simulink model "CM200C_DmaCfgAndUse"  (R2013b)
settings: Solver=ode1  StartTime=0.0  StopTime=Inf  FixedStep=0.001  RelTol=1e-3
libraries: simulink x2
(part 1 of 2)
settings Model: Creator=Keyur Patel  LastModifiedBy=CZ68DS
settings OptimizationCC: BlockReduction=off  DefaultUnderspecifiedDataType=single  OptimizeBlockIOStorage=off  BufferReuse=off  ExpressionFolding=off  LocalBlockOutputs=off  OptimizeModelRefInitCode=on  LifeSpan=Inf
settings DebuggingCC: FrameProcessingCompatibilityMsg=error
settings HardwareCC: ProdIntDivRoundTo=Zero  ProdEndianess=BigEndian  ProdHWDeviceType=Generic->Custom  TargetIntDivRoundTo=Zero  TargetEndianess=BigEndian  TargetHWDeviceType=Generic->Custom
settings RTWCC: SystemTargetFile=ert.tlc  TemplateMakefile=ert_default_tmf  Description=Embedded Coder
settings CodeAppCC: IgnoreCustomStorageClasses=off
settings ERTTargetCC: CodeReplacementLibrary=C89/C90 (ANSI)  GenerateSampleERTMain=on  ERTCustomFileTemplate=example_file_process.tlc

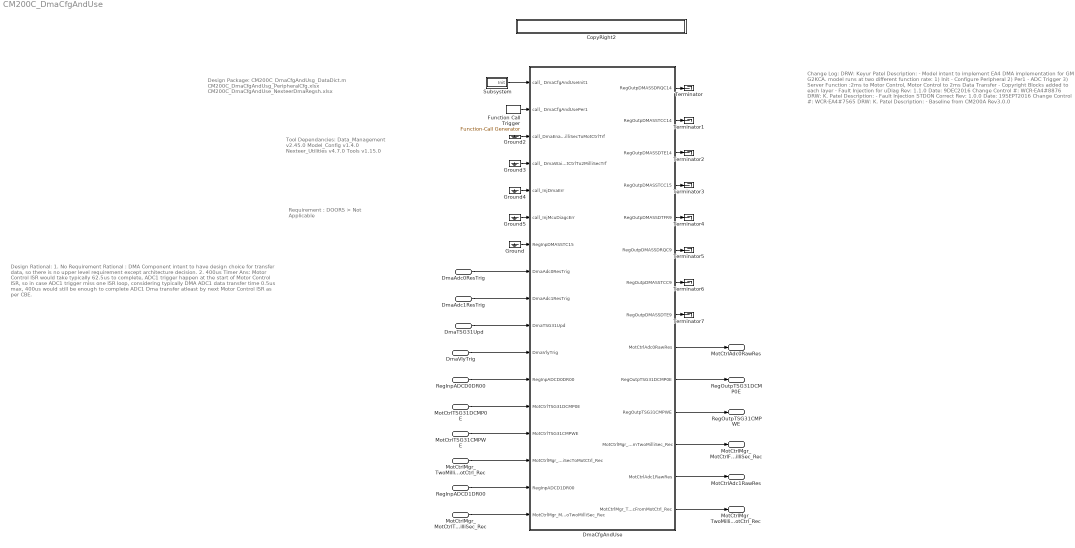
== system CM200C_DmaCfgAndUse ==
  note: Design Package:
      |
      | CM200C_DmaCfgAndUsg_DataDict.m
      | CM200C_DmaCfgAndUsg_PeripheralCfg.xlsx
      | CM200C_DmaCfgAndUse_NexteerDmaRegsh.xlsx
  note: Tool Dependancies:
      |
      | Data_Management v2.45.0
      | Model_Config v1.4.0
      | Nexteer_Utilities v4.7.0
      | Tools v1.15.0
  note: Requirement :
      |
      | DOORS > Not Applicable
  note: Change Log:
      |
      | DRW: Keyur Patel
      | Description:
      | - Model intent to implement EA4 DMA implementation for GM G2KCA.
      |    model runs at two different function rate:
      |       1) Init - Configure Peripheral
      | 	 2) Per1 - ADC Trigger
      | 	 3) Server Function :2ms to Motor Control, Motor Control to 2ms Data Transfer
      | - Copyright Blocks added to each layer
      | - Fault Injection for uDiag
      |
      | Rev: 1.1.0
      | Date: 9DEC2016
      | Change Control #: WCR-EA4#8876
      | DRW: K. Patel
      | Description:
      | - Fault Injection STDON Correct
      |
      | Rev: 1.0.0
      | Date: 19SEPT2016
      | Change Control #: WCR-EA4#7565
      | DRW: K. Patel
      | Description:
      | - Baseline from CM200A Rev3.0.0
  note: Design Rational:
      | 1. No Requirement
      | Rational :  DMA Component intent to have design choice for transfer data, so there is no upper level
      | requirement except architecture decision.
      |
      | 2. 400us Timer
      | Ans: Motor Control ISR would take typically 62.5us to complete, ADC1 trigger happen at the start of Motor
      | Control ISR, so in case ADC1  trigger miss one ISR loop, considering typically DMA ADC1 data transfer time
      | 0.5us max, 400us would still be enough to complete ADC1 Dma transfer atleast by next Motor Control
      | ISR as per CBE.
  DmaAdc0ResTrig : Inport
  DmaAdc1ResTrig : Inport  Port=2
  DmaTSG31Upd : Inport  Port=3
  DmaVlyTrig : Inport  Port=4
  RegInpADCD0DR00 : Inport  Port=5
  MotCtrlTSG31DCMP0E : Inport  Description=DMA0-3 : Source Address  Port=6
  MotCtrlTSG31CMPWE : Inport  Description=DMA0-4 : Source Address  Port=7
  MotCtrlMgr_TwoMilliSecToMotCtrl_Rec : Inport  Description=DMA1-1 : Source Address  Port=8
  RegInpADCD1DR00 : Inport  Description=DMA1-6 : Source Address  Port=9
  MotCtrlMgr_MotCtrlToTwoMilliSec_Rec : Inport  Description=DMA1-7 : Source Address  Port=10
  CopyRight2 : Subsystem  Description=|  mask(Copyright Information){none=on}
      | Copyright info block.                                               
      |                                                                     
      | Place copyright information at the top of every subsystem in design.
      mask prompts: none "No parameters"
      mask help: Place copyright information at the top of every subsystem in design.
      mask Display:
      | NxtrConf = 'Nexteer Confidential';
      | 
      | sys = bdroot; %handle for the current model ("system")
      | first = get_param(sys,'Created');
      | first = first(end-3:end);  %year is last four digits
      | 
      | last = get_param(sys,'LastModifiedDate');
      | if isempty(last)
      |     last = datestr(now,'yyyy');
      | else
      |     last = last(end-3:end);
      | end
      | 
      | if strcmp(first,last)
      |     fprintf('%s -- Copyright %s Nexteer',NxtrConf,first)
      | else
      |     fprintf('%s -- %s%s- %s Nexteer',NxtrConf,char(169),first,last)
      | end
  DmaCfgAndUse : Subsystem
  Function Call Trigger : simulink/Ports & Subsystems/Function-Call Generator  RequirementInfo="{'linktype_rmi_doors' '000089e3 (/E-STEER_New/System Specification Documents/Core Specs/Subsystem Specs/System Functions FDD/SF-46  Gross Cross Check)' '#211' 'true' 'REQ: SF046A_211' '' ; 'linktype_rmi_doors' '000089e3 (/E-STEER_New/System Specification Documents/Core Specs/Subsystem Specs/System Functions FDD/SF-46  Gross Cross Check)' '#182' 'true' 'REQ: SF046A_182' '' } %GIDa_688b36ec_1d40_4533_93c7_ec108d0c1aaf"  sample_time=0.002  numberOfIterations=1
      settings: AttributesFormatString=%<sample_time>
  Ground{,2..5} (5 alike) : Ground
  Subsystem : Subsystem
  Terminator{,1..7} (8 alike) : Terminator
  MotCtrlAdc0RawRes : Outport  Description=DMA0-1: Destination Address
  RegOutpTSG31DCMP0E : Outport  Description=DMA0-3: Destination Address  Port=2
  RegOutpTSG31CMPWE : Outport  Description=DMA0-4 : Destination Address  Port=3
  MotCtrlMgr_MotCtrlFromTwoMilliSec_Rec : Outport  Description=DMA1-1 : Destination Address  Port=4
  MotCtrlAdc1RawRes : Outport  Description=DMA1-6 : Destination Address  Port=5
  MotCtrlMgr_TwoMilliSecFromMotCtrl_Rec : Outport  Description=DMA1-7 : Destination Address  Port=6
  wires:
  Function Call Trigger/1 -> DmaCfgAndUse/2(call_ DmaCfgAndUsePer1)
  DmaCfgAndUse/1(RegOutpDMASSDRQC14) -> Terminator/1
  DmaCfgAndUse/2(RegOutpDMASSTCC14) -> Terminator1/1
  DmaCfgAndUse/3(RegOutpDMASSDTE14) -> Terminator2/1
  DmaCfgAndUse/7(RegOutpDMASSTCC9) -> Terminator6/1
  DmaCfgAndUse/6(RegOutpDMASSDRQC9) -> Terminator5/1
  DmaCfgAndUse/5(RegOutpDMASSDTFR9) -> Terminator4/1
  DmaCfgAndUse/8(RegOutpDMASSDTE9) -> Terminator7/1
  Ground/1 -> DmaCfgAndUse/7(RegInpDMASSTC15)
  DmaAdc0ResTrig/1 -> DmaCfgAndUse/8(DmaAdc0ResTrig)
  DmaAdc1ResTrig/1 -> DmaCfgAndUse/9(DmaAdc1ResTrig)
  DmaTSG31Upd/1 -> DmaCfgAndUse/10(DmaTSG31Upd)
  DmaVlyTrig/1 -> DmaCfgAndUse/11(DmaVlyTrig)
  DmaCfgAndUse/4(RegOutpDMASSTCC15) -> Terminator3/1
  RegInpADCD0DR00/1 -> DmaCfgAndUse/12(RegInpADCD0DR00)
  MotCtrlTSG31DCMP0E/1 -> DmaCfgAndUse/13(MotCtrlTSG31DCMP0E)
  MotCtrlTSG31CMPWE/1 -> DmaCfgAndUse/14(MotCtrlTSG31CMPWE)
  MotCtrlMgr_TwoMilliSecToMotCtrl_Rec/1 -> DmaCfgAndUse/15(MotCtrlMgr_TwoMilliSecToMotCtrl_Rec)
  RegInpADCD1DR00/1 -> DmaCfgAndUse/16(RegInpADCD1DR00)
  MotCtrlMgr_MotCtrlToTwoMilliSec_Rec/1 -> DmaCfgAndUse/17(MotCtrlMgr_MotCtrlToTwoMilliSec_Rec)
  DmaCfgAndUse/9(MotCtrlAdc0RawRes) -> MotCtrlAdc0RawRes/1
  DmaCfgAndUse/10(RegOutpTSG31DCMP0E) -> RegOutpTSG31DCMP0E/1
  DmaCfgAndUse/11(RegOutpTSG31CMPWE) -> RegOutpTSG31CMPWE/1
  DmaCfgAndUse/12(MotCtrlMgr_MotCtrlFromTwoMilliSec_Rec) -> MotCtrlMgr_MotCtrlFromTwoMilliSec_Rec/1
  DmaCfgAndUse/13(MotCtrlAdc1RawRes) -> MotCtrlAdc1RawRes/1
  DmaCfgAndUse/14(MotCtrlMgr_TwoMilliSecFromMotCtrl_Rec) -> MotCtrlMgr_TwoMilliSecFromMotCtrl_Rec/1
  Subsystem/1(Init) -> DmaCfgAndUse/1(call_ DmaCfgAndUseInit1)
  Ground2/1 -> DmaCfgAndUse/3(call_DmaEna2MilliSecToMotCtrlTrf)
  Ground3/1 -> DmaCfgAndUse/4(call_ DmaWaitForMotCtrlTo2MilliSecTrf)
  Ground4/1 -> DmaCfgAndUse/5(call_InjDmaErr)
  Ground5/1 -> DmaCfgAndUse/6(call_InjMcuDiagcErr)

== system CM200C_DmaCfgAndUse/CopyRight2 ==

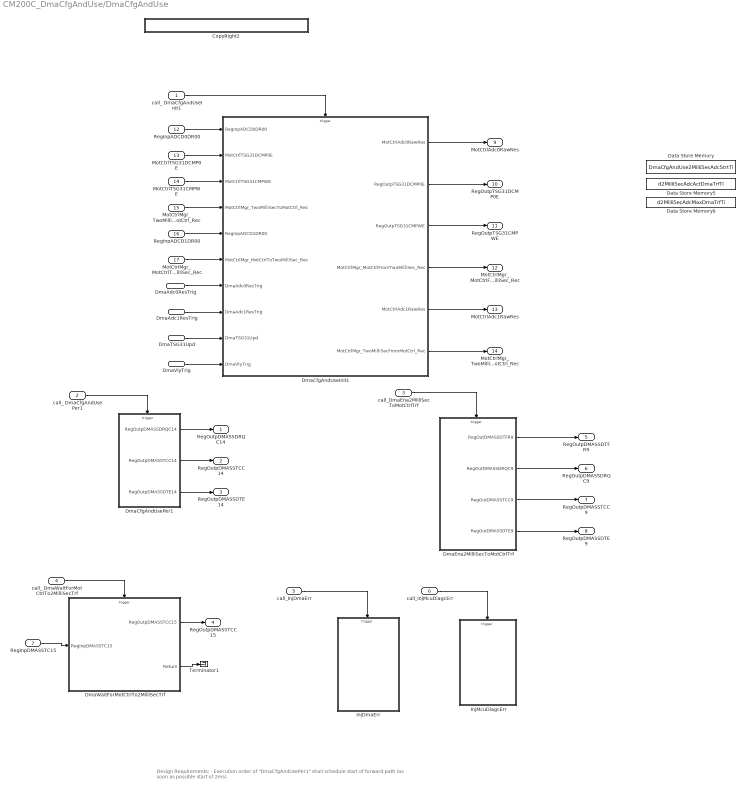
== system CM200C_DmaCfgAndUse/DmaCfgAndUse ==
  note: Design Requirements:
      |
      | - Execution order of "DmaCfgAndUsePer1" shall schedule start of forward path (as soon as possible start of 2ms).
  call_ DmaCfgAndUseInit1 : Inport
  call_ DmaCfgAndUsePer1 : Inport  Port=2
  call_DmaEna2MilliSecToMotCtrlTrf : Inport  Port=3
  call_ DmaWaitForMotCtrlTo2MilliSecTrf : Inport  Port=4
  call_InjDmaErr : Inport  Port=5
  call_InjMcuDiagcErr : Inport  Port=6
  RegInpDMASSTC15 : Inport  Port=7
  DmaAdc0ResTrig : Inport  Description=Physical Trigger : INTADCD0I3  Port=8
  DmaAdc1ResTrig : Inport  Description=Physical Trigger: INTADCD1I1  Port=9
  DmaTSG31Upd : Inport  Description=Physical Trigger: INTTSG31I11  Port=10
  DmaVlyTrig : Inport  Description=Physical Trigger: INTTSG31IVLY  Port=11
  RegInpADCD0DR00 : Inport  Port=12
  MotCtrlTSG31DCMP0E : Inport  Description=DMA0-3 : Source Address  Port=13
  MotCtrlTSG31CMPWE : Inport  Description=DMA0-4 : Source Address  Port=14
  MotCtrlMgr_TwoMilliSecToMotCtrl_Rec : Inport  Description=DMA1-1 : Source Address  Port=15
  RegInpADCD1DR00 : Inport  Description=DMA1-6 : Source Address  Port=16
  MotCtrlMgr_MotCtrlToTwoMilliSec_Rec : Inport  Description=DMA1-7 : Source Address  Port=17
  CopyRight2 : Subsystem  Description=|  mask(Copyright Information){none=on}
      | Copyright info block.                                               
      |                                                                     
      | Place copyright information at the top of every subsystem in design.
      mask prompts: none "No parameters"
      mask help: Place copyright information at the top of every subsystem in design.
      mask Display:
      | NxtrConf = 'Nexteer Confidential';
      | 
      | sys = bdroot; %handle for the current model ("system")
      | first = get_param(sys,'Created');
      | first = first(end-3:end);  %year is last four digits
      | 
      | last = get_param(sys,'LastModifiedDate');
      | if isempty(last)
      |     last = datestr(now,'yyyy');
      | else
      |     last = last(end-3:end);
      | end
      | 
      | if strcmp(first,last)
      |     fprintf('%s -- Copyright %s Nexteer',NxtrConf,first)
      | else
      |     fprintf('%s -- %s%s- %s Nexteer',NxtrConf,char(169),first,last)
      | end
  Data Store Memory : DataStoreMemory  DataStoreName=DmaCfgAndUse2MilliSecAdcStrtTi  ReadBeforeWriteMsg=warning  WriteAfterWriteMsg=warning  WriteAfterReadMsg=warning  ShowAdditionalParam=off  StateMustResolveToSignalObject=on
  Data Store Memory5 : DataStoreMemory  DataStoreName=d2MilliSecAdcActDmaTrfTi  ReadBeforeWriteMsg=warning  WriteAfterWriteMsg=warning  WriteAfterReadMsg=warning  ShowAdditionalParam=off  StateMustResolveToSignalObject=on
  Data Store Memory6 : DataStoreMemory  DataStoreName=d2MilliSecAdcMaxDmaTrfTi  ReadBeforeWriteMsg=warning  WriteAfterWriteMsg=warning  WriteAfterReadMsg=warning  ShowAdditionalParam=off  StateMustResolveToSignalObject=on
  DmaCfgAndUseInit1 : Subsystem  TreatAsAtomicUnit=on
  DmaCfgAndUsePer1 : Subsystem  TreatAsAtomicUnit=on
  DmaEna2MilliSecToMotCtrlTrf : Subsystem  TreatAsAtomicUnit=on
  DmaWaitForMotCtrlTo2MilliSecTrf : Subsystem  TreatAsAtomicUnit=on
  InjDmaErr : Subsystem  TreatAsAtomicUnit=on
  InjMcuDiagcErr : Subsystem  TreatAsAtomicUnit=on
  Terminator1 : Terminator
  RegOutpDMASSDRQC14 : Outport
  RegOutpDMASSTCC14 : Outport  Port=2
  RegOutpDMASSDTE14 : Outport  Port=3
  RegOutpDMASSTCC15 : Outport  Port=4
  RegOutpDMASSDTFR9 : Outport  Port=5
  RegOutpDMASSDRQC9 : Outport  Port=6
  RegOutpDMASSTCC9 : Outport  Port=7
  RegOutpDMASSDTE9 : Outport  Port=8
  MotCtrlAdc0RawRes : Outport  Description=DMA0-1: Destination Address  Port=9
  RegOutpTSG31DCMP0E : Outport  Description=DMA0-3: Destination Address  Port=10
  RegOutpTSG31CMPWE : Outport  Description=DMA0-4 : Destination Address  Port=11
  MotCtrlMgr_MotCtrlFromTwoMilliSec_Rec : Outport  Description=DMA1-1 : Destination Address  Port=12
  MotCtrlAdc1RawRes : Outport  Description=DMA1-6 : Destination Address  Port=13
  MotCtrlMgr_TwoMilliSecFromMotCtrl_Rec : Outport  Description=DMA1-7 : Destination Address  Port=14
  wires:
  call_ DmaCfgAndUseInit1/1 -> DmaCfgAndUseInit1/Trigger
  call_ DmaCfgAndUsePer1/1 -> DmaCfgAndUsePer1/Trigger
  call_ DmaWaitForMotCtrlTo2MilliSecTrf/1 -> DmaWaitForMotCtrlTo2MilliSecTrf/Trigger
  call_DmaEna2MilliSecToMotCtrlTrf/1 -> DmaEna2MilliSecToMotCtrlTrf/Trigger
  DmaCfgAndUsePer1/3(RegOutpDMASSDTE14) -> RegOutpDMASSDTE14/1
  DmaCfgAndUsePer1/2(RegOutpDMASSTCC14) -> RegOutpDMASSTCC14/1
  DmaCfgAndUsePer1/1(RegOutpDMASSDRQC14) -> RegOutpDMASSDRQC14/1
  DmaWaitForMotCtrlTo2MilliSecTrf/1(RegOutpDMASSTCC15) -> RegOutpDMASSTCC15/1
  DmaEna2MilliSecToMotCtrlTrf/2(RegOutDMASSDRQC9) -> RegOutpDMASSDRQC9/1
  DmaEna2MilliSecToMotCtrlTrf/4(RegOutDMASSDTE9) -> RegOutpDMASSDTE9/1
  DmaEna2MilliSecToMotCtrlTrf/3(RegOutDMASSTCC9) -> RegOutpDMASSTCC9/1
  DmaEna2MilliSecToMotCtrlTrf/1(RegOutDMASSDTFR9) -> RegOutpDMASSDTFR9/1
  RegInpDMASSTC15/1 -> DmaWaitForMotCtrlTo2MilliSecTrf/1(RegInpDMASSTC15)
  MotCtrlMgr_MotCtrlToTwoMilliSec_Rec/1 -> DmaCfgAndUseInit1/6(MotCtrlMgr_MotCtrlToTwoMilliSec_Rec)
  RegInpADCD0DR00/1 -> DmaCfgAndUseInit1/1(RegInpADCD0DR00)
  RegInpADCD1DR00/1 -> DmaCfgAndUseInit1/5(RegInpADCD1DR00)
  MotCtrlMgr_TwoMilliSecToMotCtrl_Rec/1 -> DmaCfgAndUseInit1/4(MotCtrlMgr_TwoMilliSecToMotCtrl_Rec)
  MotCtrlTSG31DCMP0E/1 -> DmaCfgAndUseInit1/2(MotCtrlTSG31DCMP0E)
  MotCtrlTSG31CMPWE/1 -> DmaCfgAndUseInit1/3(MotCtrlTSG31CMPWE)
  DmaAdc0ResTrig/1 -> DmaCfgAndUseInit1/7(DmaAdc0ResTrig)
  DmaAdc1ResTrig/1 -> DmaCfgAndUseInit1/8(DmaAdc1ResTrig)
  DmaTSG31Upd/1 -> DmaCfgAndUseInit1/9(DmaTSG31Upd)
  DmaVlyTrig/1 -> DmaCfgAndUseInit1/10(DmaVlyTrig)
  DmaWaitForMotCtrlTo2MilliSecTrf/2(Return) -> Terminator1/1
  DmaCfgAndUseInit1/1(MotCtrlAdc0RawRes) -> MotCtrlAdc0RawRes/1
  DmaCfgAndUseInit1/6(MotCtrlMgr_TwoMilliSecFromMotCtrl_Rec) -> MotCtrlMgr_TwoMilliSecFromMotCtrl_Rec/1
  DmaCfgAndUseInit1/2(RegOutpTSG31DCMP0E) -> RegOutpTSG31DCMP0E/1
  DmaCfgAndUseInit1/3(RegOutpTSG31CMPWE) -> RegOutpTSG31CMPWE/1
  DmaCfgAndUseInit1/5(MotCtrlAdc1RawRes) -> MotCtrlAdc1RawRes/1
  DmaCfgAndUseInit1/4(MotCtrlMgr_MotCtrlFromTwoMilliSec_Rec) -> MotCtrlMgr_MotCtrlFromTwoMilliSec_Rec/1
  call_InjDmaErr/1 -> InjDmaErr/Trigger
  call_InjMcuDiagcErr/1 -> InjMcuDiagcErr/Trigger

== system CM200C_DmaCfgAndUse/Subsystem ==
  CopyRight2 : Subsystem  Description=|  mask(Copyright Information){none=on}
      | Copyright info block.                                               
      |                                                                     
      | Place copyright information at the top of every subsystem in design.
      mask prompts: none "No parameters"
      mask help: Place copyright information at the top of every subsystem in design.
      mask Display:
      | NxtrConf = 'Nexteer Confidential';
      | 
      | sys = bdroot; %handle for the current model ("system")
      | first = get_param(sys,'Created');
      | first = first(end-3:end);  %year is last four digits
      | 
      | last = get_param(sys,'LastModifiedDate');
      | if isempty(last)
      |     last = datestr(now,'yyyy');
      | else
      |     last = last(end-3:end);
      | end
      | 
      | if strcmp(first,last)
      |     fprintf('%s -- Copyright %s Nexteer',NxtrConf,first)
      | else
      |     fprintf('%s -- %s%s- %s Nexteer',NxtrConf,char(169),first,last)
      | end
  Enabled Subsystem : Subsystem  TreatAsAtomicUnit=on
  Step : Step  Before=1  After=0  SampleTime=0
  Init : Outport
  wires:
  Enabled Subsystem/1(Init) -> Init/1
  Step/1 -> Enabled Subsystem/Enable

== system CM200C_DmaCfgAndUse/DmaCfgAndUse/CopyRight2 ==

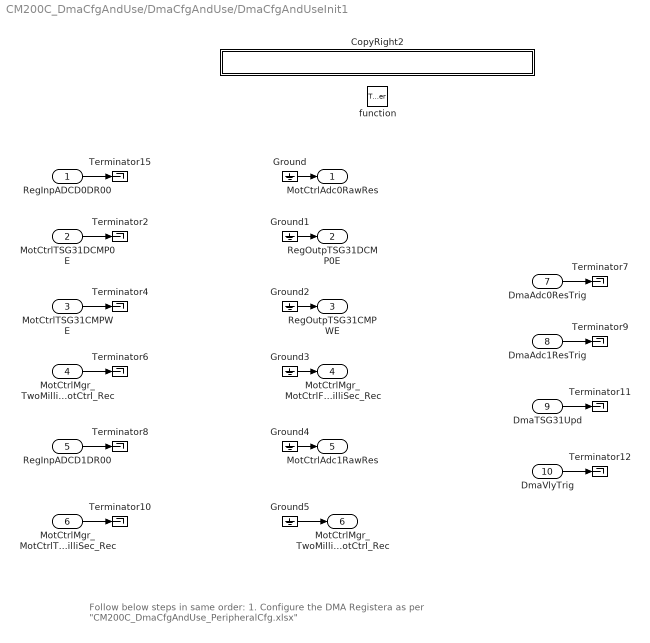
== system CM200C_DmaCfgAndUse/DmaCfgAndUse/DmaCfgAndUseInit1 ==
  note: Follow below steps in same order:
      |
      | 1. Configure the DMA Registera as per  "CM200C_DmaCfgAndUse_PeripheralCfg.xlsx"
  RegInpADCD0DR00 : Inport
      settings: AttributesFormatString=DMA0-1 : Source Address
  MotCtrlTSG31DCMP0E : Inport  Port=2
      settings: AttributesFormatString=DMA0-3 : Source Address
  MotCtrlTSG31CMPWE : Inport  Port=3
      settings: AttributesFormatString=DMA0-4 : Source Address
  MotCtrlMgr_TwoMilliSecToMotCtrl_Rec : Inport  Port=4
      settings: AttributesFormatString=DMA1-1 : Source Address
  RegInpADCD1DR00 : Inport  Port=5
      settings: AttributesFormatString=DMA1-6 : Source Address
  MotCtrlMgr_MotCtrlToTwoMilliSec_Rec : Inport  Port=6
      settings: AttributesFormatString=DMA1-7 : Source Address
  DmaAdc0ResTrig : Inport  Description=Physical Trigger : INTADCD0I3  Port=7
      settings: AttributesFormatString=%<Description>
  DmaAdc1ResTrig : Inport  Description=Physical Trigger: INTADCD1I1  Port=8
      settings: AttributesFormatString=%<Description>
  DmaTSG31Upd : Inport  Description=Physical Trigger: INTTSG31I11  Port=9
      settings: AttributesFormatString=%<Description>
  DmaVlyTrig : Inport  Description=Physical Trigger: INTTSG31VI  Port=10
      settings: AttributesFormatString=%<Description>
  function : TriggerPort  TriggerType=function-call
  CopyRight2 : Subsystem  Description=|  mask(Copyright Information){none=on}
      | Copyright info block.                                               
      |                                                                     
      | Place copyright information at the top of every subsystem in design.
      mask prompts: none "No parameters"
      mask help: Place copyright information at the top of every subsystem in design.
      mask Display:
      | NxtrConf = 'Nexteer Confidential';
      | 
      | sys = bdroot; %handle for the current model ("system")
      | first = get_param(sys,'Created');
      | first = first(end-3:end);  %year is last four digits
      | 
      | last = get_param(sys,'LastModifiedDate');
      | if isempty(last)
      |     last = datestr(now,'yyyy');
      | else
      |     last = last(end-3:end);
      | end
      | 
      | if strcmp(first,last)
      |     fprintf('%s -- Copyright %s Nexteer',NxtrConf,first)
      | else
      |     fprintf('%s -- %s%s- %s Nexteer',NxtrConf,char(169),first,last)
      | end
  Ground{,1..5} (6 alike) : Ground
  Terminator{2,4,6..12,15} (10 alike) : Terminator
  MotCtrlAdc0RawRes : Outport  Description=DMA0-1: Destination Address
      settings: AttributesFormatString=%<Description>
  RegOutpTSG31DCMP0E : Outport  Description=DMA0-3: Destination Address  Port=2
      settings: AttributesFormatString=%<Description>
  RegOutpTSG31CMPWE : Outport  Description=DMA0-4 : Destination Address  Port=3
      settings: AttributesFormatString=%<Description>
  MotCtrlMgr_MotCtrlFromTwoMilliSec_Rec : Outport  Description=DMA1-1 : Destination Address  Port=4
      settings: AttributesFormatString=%<Description>
  MotCtrlAdc1RawRes : Outport  Description=DMA1-6 : Destination Address  Port=5
      settings: AttributesFormatString=%<Description>
  MotCtrlMgr_TwoMilliSecFromMotCtrl_Rec : Outport  Description=DMA1-7 : Destination Address  Port=6
      settings: AttributesFormatString=%<Description>
  wires:
  RegInpADCD0DR00/1 -> Terminator15/1
  MotCtrlTSG31DCMP0E/1 -> Terminator2/1
  MotCtrlTSG31CMPWE/1 -> Terminator4/1
  MotCtrlMgr_TwoMilliSecToMotCtrl_Rec/1 -> Terminator6/1
  RegInpADCD1DR00/1 -> Terminator8/1
  MotCtrlMgr_MotCtrlToTwoMilliSec_Rec/1 -> Terminator10/1
  Ground/1 -> MotCtrlAdc0RawRes/1
  Ground1/1 -> RegOutpTSG31DCMP0E/1
  Ground2/1 -> RegOutpTSG31CMPWE/1
  Ground3/1 -> MotCtrlMgr_MotCtrlFromTwoMilliSec_Rec/1
  Ground4/1 -> MotCtrlAdc1RawRes/1
  Ground5/1 -> MotCtrlMgr_TwoMilliSecFromMotCtrl_Rec/1
  DmaAdc0ResTrig/1 -> Terminator7/1
  DmaAdc1ResTrig/1 -> Terminator9/1
  DmaTSG31Upd/1 -> Terminator11/1
  DmaVlyTrig/1 -> Terminator12/1

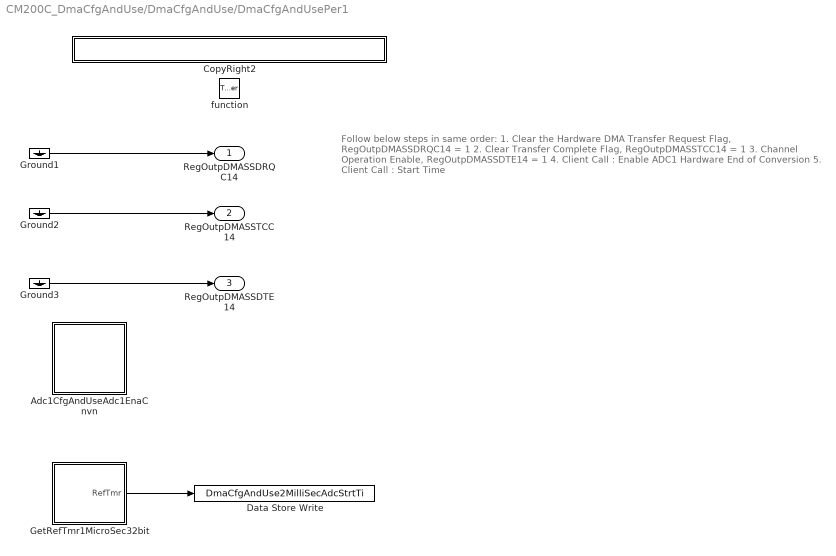
== system CM200C_DmaCfgAndUse/DmaCfgAndUse/DmaCfgAndUsePer1 ==
  note: Follow below steps in same order:
      |
      | 1. Clear the Hardware DMA Transfer Request Flag, RegOutpDMASSDRQC14 = 1
      | 2. Clear Transfer Complete Flag, RegOutpDMASSTCC14 = 1
      | 3. Channel Operation Enable, RegOutpDMASSDTE14 = 1
      | 4. Client Call : Enable ADC1 Hardware End of Conversion
      | 5. Client Call : Start Time
  function : TriggerPort  TriggerType=function-call
  Adc1CfgAndUseAdc1EnaCnvn : Subsystem
      settings: AttributesFormatString=Client Call : Enable ADC1 Hardware End of Conversion
  CopyRight2 : Subsystem  Description=|  mask(Copyright Information){none=on}
      | Copyright info block.                                               
      |                                                                     
      | Place copyright information at the top of every subsystem in design.
      mask prompts: none "No parameters"
      mask help: Place copyright information at the top of every subsystem in design.
      mask Display:
      | NxtrConf = 'Nexteer Confidential';
      | 
      | sys = bdroot; %handle for the current model ("system")
      | first = get_param(sys,'Created');
      | first = first(end-3:end);  %year is last four digits
      | 
      | last = get_param(sys,'LastModifiedDate');
      | if isempty(last)
      |     last = datestr(now,'yyyy');
      | else
      |     last = last(end-3:end);
      | end
      | 
      | if strcmp(first,last)
      |     fprintf('%s -- Copyright %s Nexteer',NxtrConf,first)
      | else
      |     fprintf('%s -- %s%s- %s Nexteer',NxtrConf,char(169),first,last)
      | end
  Data Store Write : DataStoreWrite  DataStoreName=DmaCfgAndUse2MilliSecAdcStrtTi
  GetRefTmr1MicroSec32bit : Subsystem
      settings: AttributesFormatString=Client Call : Start Time
  Ground1 : Ground
  Ground2 : Ground
  Ground3 : Ground
  RegOutpDMASSDRQC14 : Outport
  RegOutpDMASSTCC14 : Outport  Port=2
  RegOutpDMASSDTE14 : Outport  Port=3
  wires:
  Ground1/1 -> RegOutpDMASSDRQC14/1
  Ground2/1 -> RegOutpDMASSTCC14/1
  Ground3/1 -> RegOutpDMASSDTE14/1
  GetRefTmr1MicroSec32bit/1(RefTmr) -> Data Store Write/1

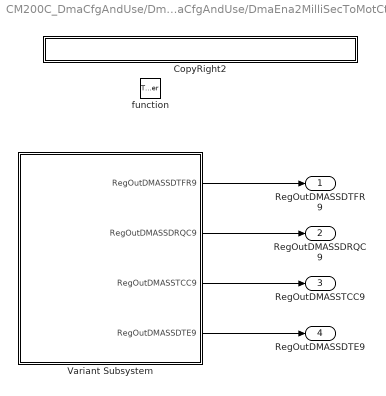
== system CM200C_DmaCfgAndUse/DmaCfgAndUse/DmaEna2MilliSecToMotCtrlTrf ==
  function : TriggerPort  TriggerType=function-call
  CopyRight2 : Subsystem  Description=|  mask(Copyright Information){none=on}
      | Copyright info block.                                               
      |                                                                     
      | Place copyright information at the top of every subsystem in design.
      mask prompts: none "No parameters"
      mask help: Place copyright information at the top of every subsystem in design.
      mask Display:
      | NxtrConf = 'Nexteer Confidential';
      | 
      | sys = bdroot; %handle for the current model ("system")
      | first = get_param(sys,'Created');
      | first = first(end-3:end);  %year is last four digits
      | 
      | last = get_param(sys,'LastModifiedDate');
      | if isempty(last)
      |     last = datestr(now,'yyyy');
      | else
      |     last = last(end-3:end);
      | end
      | 
      | if strcmp(first,last)
      |     fprintf('%s -- Copyright %s Nexteer',NxtrConf,first)
      | else
      |     fprintf('%s -- %s%s- %s Nexteer',NxtrConf,char(169),first,last)
      | end
  Variant Subsystem : Subsystem  Variant=on
      settings: AttributesFormatString=%<VariantControl>
  RegOutDMASSDTFR9 : Outport
  RegOutDMASSDRQC9 : Outport  Port=2
  RegOutDMASSTCC9 : Outport  Port=3
  RegOutDMASSDTE9 : Outport  Port=4
  wires:
  Variant Subsystem/2(RegOutDMASSDRQC9) -> RegOutDMASSDRQC9/1
  Variant Subsystem/1(RegOutDMASSDTFR9) -> RegOutDMASSDTFR9/1
  Variant Subsystem/3(RegOutDMASSTCC9) -> RegOutDMASSTCC9/1
  Variant Subsystem/4(RegOutDMASSDTE9) -> RegOutDMASSDTE9/1

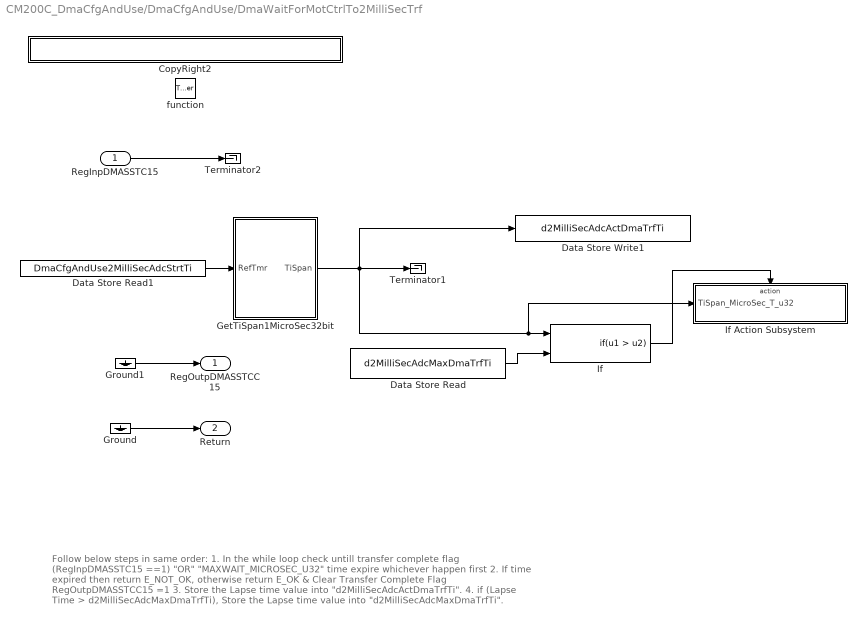
== system CM200C_DmaCfgAndUse/DmaCfgAndUse/DmaWaitForMotCtrlTo2MilliSecTrf ==
  note: Follow below steps in same order:
      |
      | 1. In the while loop check untill transfer complete flag (RegInpDMASSTC15 ==1) "OR" "MAXWAIT_MICROSEC_U32" time expire whichever happen first
      | 2. If time expired then return E_NOT_OK,
      |     otherwise return E_OK & Clear Transfer Complete Flag RegOutpDMASSTCC15 =1
      | 3. Store the Lapse time value into "d2MilliSecAdcActDmaTrfTi".
      | 4. if (Lapse Time > d2MilliSecAdcMaxDmaTrfTi), Store the Lapse time value into "d2MilliSecAdcMaxDmaTrfTi".
  RegInpDMASSTC15 : Inport
      settings: AttributesFormatString=Transfer Complete Flag Status Check
  function : TriggerPort  TriggerType=function-call
  CopyRight2 : Subsystem  Description=|  mask(Copyright Information){none=on}
      | Copyright info block.                                               
      |                                                                     
      | Place copyright information at the top of every subsystem in design.
      mask prompts: none "No parameters"
      mask help: Place copyright information at the top of every subsystem in design.
      mask Display:
      | NxtrConf = 'Nexteer Confidential';
      | 
      | sys = bdroot; %handle for the current model ("system")
      | first = get_param(sys,'Created');
      | first = first(end-3:end);  %year is last four digits
      | 
      | last = get_param(sys,'LastModifiedDate');
      | if isempty(last)
      |     last = datestr(now,'yyyy');
      | else
      |     last = last(end-3:end);
      | end
      | 
      | if strcmp(first,last)
      |     fprintf('%s -- Copyright %s Nexteer',NxtrConf,first)
      | else
      |     fprintf('%s -- %s%s- %s Nexteer',NxtrConf,char(169),first,last)
      | end
  Data Store Read : DataStoreRead  DataStoreName=d2MilliSecAdcMaxDmaTrfTi
  Data Store Read1 : DataStoreRead  DataStoreName=DmaCfgAndUse2MilliSecAdcStrtTi
  Data Store Write1 : DataStoreWrite  DataStoreName=d2MilliSecAdcActDmaTrfTi
  GetTiSpan1MicroSec32bit : Subsystem
  Ground : Ground
  Ground1 : Ground
  If : If  NumInputs=2  IfExpression=u1 > u2  ShowElse=off
  If Action Subsystem : Subsystem  TreatAsAtomicUnit=on
  Terminator1 : Terminator
      settings: Description=TiSpan_MicroSec_T_u32  AttributesFormatString=%<Description>
  Terminator2 : Terminator
  RegOutpDMASSTCC15 : Outport
  Return : Outport  Port=2
  wires:
  Ground1/1 -> RegOutpDMASSTCC15/1
  RegInpDMASSTC15/1 -> Terminator2/1
  Ground/1 -> Return/1
  Data Store Read1/1 -> GetTiSpan1MicroSec32bit/1(RefTmr)
  GetTiSpan1MicroSec32bit/1(TiSpan) -> Data Store Write1/1, If Action Subsystem/1(TiSpan_MicroSec_T_u32), If/1, Terminator1/1
  If/1 -> If Action Subsystem/Action
  Data Store Read/1 -> If/2

== system CM200C_DmaCfgAndUse/DmaCfgAndUse/InjDmaErr ==
  function : TriggerPort  TriggerType=function-call
  CopyRight2 : Subsystem  Description=|  mask(Copyright Information){none=on}
      | Copyright info block.                                               
      |                                                                     
      | Place copyright information at the top of every subsystem in design.
      mask prompts: none "No parameters"
      mask help: Place copyright information at the top of every subsystem in design.
      mask Display:
      | NxtrConf = 'Nexteer Confidential';
      | 
      | sys = bdroot; %handle for the current model ("system")
      | first = get_param(sys,'Created');
      | first = first(end-3:end);  %year is last four digits
      | 
      | last = get_param(sys,'LastModifiedDate');
      | if isempty(last)
      |     last = datestr(now,'yyyy');
      | else
      |     last = last(end-3:end);
      | end
      | 
      | if strcmp(first,last)
      |     fprintf('%s -- Copyright %s Nexteer',NxtrConf,first)
      | else
      |     fprintf('%s -- %s%s- %s Nexteer',NxtrConf,char(169),first,last)
      | end
  Variant Subsystem : Subsystem  Variant=on

== system CM200C_DmaCfgAndUse/DmaCfgAndUse/InjMcuDiagcErr ==
  function : TriggerPort  TriggerType=function-call
  CopyRight2 : Subsystem  Description=|  mask(Copyright Information){none=on}
      | Copyright info block.                                               
      |                                                                     
      | Place copyright information at the top of every subsystem in design.
      mask prompts: none "No parameters"
      mask help: Place copyright information at the top of every subsystem in design.
      mask Display:
      | NxtrConf = 'Nexteer Confidential';
      | 
      | sys = bdroot; %handle for the current model ("system")
      | first = get_param(sys,'Created');
      | first = first(end-3:end);  %year is last four digits
      | 
      | last = get_param(sys,'LastModifiedDate');
      | if isempty(last)
      |     last = datestr(now,'yyyy');
      | else
      |     last = last(end-3:end);
      | end
      | 
      | if strcmp(first,last)
      |     fprintf('%s -- Copyright %s Nexteer',NxtrConf,first)
      | else
      |     fprintf('%s -- %s%s- %s Nexteer',NxtrConf,char(169),first,last)
      | end
  Variant Subsystem : Subsystem  Variant=on

== system CM200C_DmaCfgAndUse/Subsystem/CopyRight2 ==

== system CM200C_DmaCfgAndUse/Subsystem/Enabled Subsystem ==
  Enable : EnablePort
  CopyRight2 : Subsystem  Description=|  mask(Copyright Information){none=on}
      | Copyright info block.                                               
      |                                                                     
      | Place copyright information at the top of every subsystem in design.
      mask prompts: none "No parameters"
      mask help: Place copyright information at the top of every subsystem in design.
      mask Display:
      | NxtrConf = 'Nexteer Confidential';
      | 
      | sys = bdroot; %handle for the current model ("system")
      | first = get_param(sys,'Created');
      | first = first(end-3:end);  %year is last four digits
      | 
      | last = get_param(sys,'LastModifiedDate');
      | if isempty(last)
      |     last = datestr(now,'yyyy');
      | else
      |     last = last(end-3:end);
      | end
      | 
      | if strcmp(first,last)
      |     fprintf('%s -- Copyright %s Nexteer',NxtrConf,first)
      | else
      |     fprintf('%s -- %s%s- %s Nexteer',NxtrConf,char(169),first,last)
      | end
  Function Call Trigger : simulink/Ports & Subsystems/Function-Call Generator  RequirementInfo="{'linktype_rmi_doors' '000089e3 (/E-STEER_New/System Specification Documents/Core Specs/Subsystem Specs/System Functions FDD/SF-46  Gross Cross Check)' '#211' 'true' 'REQ: SF046A_211' '' ; 'linktype_rmi_doors' '000089e3 (/E-STEER_New/System Specification Documents/Core Specs/Subsystem Specs/System Functions FDD/SF-46  Gross Cross Check)' '#182' 'true' 'REQ: SF046A_182' '' } %GIDa_cf5bacff_48a9_4312_b446_700ab36e3d94"  sample_time=0.002  numberOfIterations=1
      settings: AttributesFormatString=%<sample_time>
  Init : Outport
  wires:
  Function Call Trigger/1 -> Init/1

== system CM200C_DmaCfgAndUse/DmaCfgAndUse/DmaCfgAndUseInit1/CopyRight2 ==

== system CM200C_DmaCfgAndUse/DmaCfgAndUse/DmaCfgAndUsePer1/Adc1CfgAndUseAdc1EnaCnvn ==
  CopyRight2 : Subsystem  Description=|  mask(Copyright Information){none=on}
      | Copyright info block.                                               
      |                                                                     
      | Place copyright information at the top of every subsystem in design.
      mask prompts: none "No parameters"
      mask help: Place copyright information at the top of every subsystem in design.
      mask Display:
      | NxtrConf = 'Nexteer Confidential';
      | 
      | sys = bdroot; %handle for the current model ("system")
      | first = get_param(sys,'Created');
      | first = first(end-3:end);  %year is last four digits
      | 
      | last = get_param(sys,'LastModifiedDate');
      | if isempty(last)
      |     last = datestr(now,'yyyy');
      | else
      |     last = last(end-3:end);
      | end
      | 
      | if strcmp(first,last)
      |     fprintf('%s -- Copyright %s Nexteer',NxtrConf,first)
      | else
      |     fprintf('%s -- %s%s- %s Nexteer',NxtrConf,char(169),first,last)
      | end

== system CM200C_DmaCfgAndUse/DmaCfgAndUse/DmaCfgAndUsePer1/CopyRight2 ==

== system CM200C_DmaCfgAndUse/DmaCfgAndUse/DmaCfgAndUsePer1/GetRefTmr1MicroSec32bit ==
  CopyRight2 : Subsystem  Description=|  mask(Copyright Information){none=on}
      | Copyright info block.                                               
      |                                                                     
      | Place copyright information at the top of every subsystem in design.
      mask prompts: none "No parameters"
      mask help: Place copyright information at the top of every subsystem in design.
      mask Display:
      | NxtrConf = 'Nexteer Confidential';
      | 
      | sys = bdroot; %handle for the current model ("system")
      | first = get_param(sys,'Created');
      | first = first(end-3:end);  %year is last four digits
      | 
      | last = get_param(sys,'LastModifiedDate');
      | if isempty(last)
      |     last = datestr(now,'yyyy');
      | else
      |     last = last(end-3:end);
      | end
      | 
      | if strcmp(first,last)
      |     fprintf('%s -- Copyright %s Nexteer',NxtrConf,first)
      | else
      |     fprintf('%s -- %s%s- %s Nexteer',NxtrConf,char(169),first,last)
      | end
  Ground : Ground
  RefTmr : Outport
  wires:
  Ground/1 -> RefTmr/1

== system CM200C_DmaCfgAndUse/DmaCfgAndUse/DmaEna2MilliSecToMotCtrlTrf/CopyRight2 ==

== system CM200C_DmaCfgAndUse/DmaCfgAndUse/DmaEna2MilliSecToMotCtrlTrf/Variant Subsystem ==
  note: 1) Add Subsystem or Model blocks as valid variant choices.
      | 2) You cannot connect blocks at this level. At simulation, connectivity is automatically
      | determined, based on the active variant and port name matching.
  ErrInj : Subsystem  VariantControl=MCUDIAGCERRINJ == STD_ON
  NoErrInj : Subsystem  VariantControl=MCUDIAGCERRINJ == STD_OFF
  RegOutDMASSDTFR9 : Outport
  RegOutDMASSDRQC9 : Outport  Port=2
  RegOutDMASSTCC9 : Outport  Port=3
  RegOutDMASSDTE9 : Outport  Port=4

== system CM200C_DmaCfgAndUse/DmaCfgAndUse/DmaWaitForMotCtrlTo2MilliSecTrf/CopyRight2 ==

== system CM200C_DmaCfgAndUse/DmaCfgAndUse/DmaWaitForMotCtrlTo2MilliSecTrf/GetTiSpan1MicroSec32bit ==
  RefTmr : Inport
  CopyRight2 : Subsystem  Description=|  mask(Copyright Information){none=on}
      | Copyright info block.                                               
      |                                                                     
      | Place copyright information at the top of every subsystem in design.
      mask prompts: none "No parameters"
      mask help: Place copyright information at the top of every subsystem in design.
      mask Display:
      | NxtrConf = 'Nexteer Confidential';
      | 
      | sys = bdroot; %handle for the current model ("system")
      | first = get_param(sys,'Created');
      | first = first(end-3:end);  %year is last four digits
      | 
      | last = get_param(sys,'LastModifiedDate');
      | if isempty(last)
      |     last = datestr(now,'yyyy');
      | else
      |     last = last(end-3:end);
      | end
      | 
      | if strcmp(first,last)
      |     fprintf('%s -- Copyright %s Nexteer',NxtrConf,first)
      | else
      |     fprintf('%s -- %s%s- %s Nexteer',NxtrConf,char(169),first,last)
      | end
  Ground : Ground
  TiSpan : Outport
  wires:
  Ground/1 -> TiSpan/1

== system CM200C_DmaCfgAndUse/DmaCfgAndUse/DmaWaitForMotCtrlTo2MilliSecTrf/If Action Subsystem ==
  TiSpan_MicroSec_T_u32 : Inport
  Action Port : ActionPort  ActionType=then
  CopyRight2 : Subsystem  Description=|  mask(Copyright Information){none=on}
      | Copyright info block.                                               
      |                                                                     
      | Place copyright information at the top of every subsystem in design.
      mask prompts: none "No parameters"
      mask help: Place copyright information at the top of every subsystem in design.
      mask Display:
      | NxtrConf = 'Nexteer Confidential';
      | 
      | sys = bdroot; %handle for the current model ("system")
      | first = get_param(sys,'Created');
      | first = first(end-3:end);  %year is last four digits
      | 
      | last = get_param(sys,'LastModifiedDate');
      | if isempty(last)
      |     last = datestr(now,'yyyy');
      | else
      |     last = last(end-3:end);
      | end
      | 
      | if strcmp(first,last)
      |     fprintf('%s -- Copyright %s Nexteer',NxtrConf,first)
      | else
      |     fprintf('%s -- %s%s- %s Nexteer',NxtrConf,char(169),first,last)
      | end
  Data Store Write : DataStoreWrite  DataStoreName=d2MilliSecAdcMaxDmaTrfTi
  wires:
  TiSpan_MicroSec_T_u32/1 -> Data Store Write/1

== system CM200C_DmaCfgAndUse/DmaCfgAndUse/InjDmaErr/CopyRight2 ==

== system CM200C_DmaCfgAndUse/DmaCfgAndUse/InjDmaErr/Variant Subsystem ==
  note: 1) Add Subsystem or Model blocks as valid variant choices.
      | 2) You cannot connect blocks at this level. At simulation, connectivity is automatically
      | determined, based on the active variant and port name matching.
  ErrInj : Subsystem  VariantControl=MCUDIAGCERRINJ == STD_ON

== system CM200C_DmaCfgAndUse/DmaCfgAndUse/InjMcuDiagcErr/CopyRight2 ==

== system CM200C_DmaCfgAndUse/DmaCfgAndUse/InjMcuDiagcErr/Variant Subsystem ==
  note: 1) Add Subsystem or Model blocks as valid variant choices.
      | 2) You cannot connect blocks at this level. At simulation, connectivity is automatically
      | determined, based on the active variant and port name matching.
  ErrInj : Subsystem  VariantControl=MCUDIAGCERRINJ == STD_ON

== system CM200C_DmaCfgAndUse/Subsystem/Enabled Subsystem/CopyRight2 ==

== system CM200C_DmaCfgAndUse/DmaCfgAndUse/DmaCfgAndUsePer1/Adc1CfgAndUseAdc1EnaCnvn/CopyRight2 ==

== system CM200C_DmaCfgAndUse/DmaCfgAndUse/DmaCfgAndUsePer1/GetRefTmr1MicroSec32bit/CopyRight2 ==

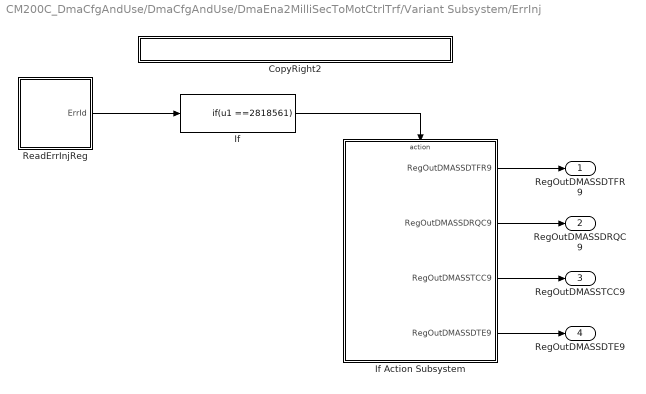
== system CM200C_DmaCfgAndUse/DmaCfgAndUse/DmaEna2MilliSecToMotCtrlTrf/Variant Subsystem/ErrInj ==
  CopyRight2 : Subsystem  Description=|  mask(Copyright Information){none=on}
      | Copyright info block.                                               
      |                                                                     
      | Place copyright information at the top of every subsystem in design.
      mask prompts: none "No parameters"
      mask help: Place copyright information at the top of every subsystem in design.
      mask Display:
      | NxtrConf = 'Nexteer Confidential';
      | 
      | sys = bdroot; %handle for the current model ("system")
      | first = get_param(sys,'Created');
      | first = first(end-3:end);  %year is last four digits
      | 
      | last = get_param(sys,'LastModifiedDate');
      | if isempty(last)
      |     last = datestr(now,'yyyy');
      | else
      |     last = last(end-3:end);
      | end
      | 
      | if strcmp(first,last)
      |     fprintf('%s -- Copyright %s Nexteer',NxtrConf,first)
      | else
      |     fprintf('%s -- %s%s- %s Nexteer',NxtrConf,char(169),first,last)
      | end
  If : If  Description=Err ID - 0x002B0201  IfExpression=u1 ==2818561  ShowElse=off
      settings: AttributesFormatString=|
      | %<IfExpression>
      | %<Description>
  If Action Subsystem : Subsystem  TreatAsAtomicUnit=on
  ReadErrInjReg : Subsystem
      settings: AttributesFormatString=Client Call : Read the Fault Injection Register
  RegOutDMASSDTFR9 : Outport
  RegOutDMASSDRQC9 : Outport  Port=2
  RegOutDMASSTCC9 : Outport  Port=3
  RegOutDMASSDTE9 : Outport  Port=4
  wires:
  ReadErrInjReg/1(ErrId) -> If/1
  If/1 -> If Action Subsystem/Action
  If Action Subsystem/3(RegOutDMASSTCC9) -> RegOutDMASSTCC9/1
  If Action Subsystem/1(RegOutDMASSDTFR9) -> RegOutDMASSDTFR9/1
  If Action Subsystem/2(RegOutDMASSDRQC9) -> RegOutDMASSDRQC9/1
  If Action Subsystem/4(RegOutDMASSDTE9) -> RegOutDMASSDTE9/1

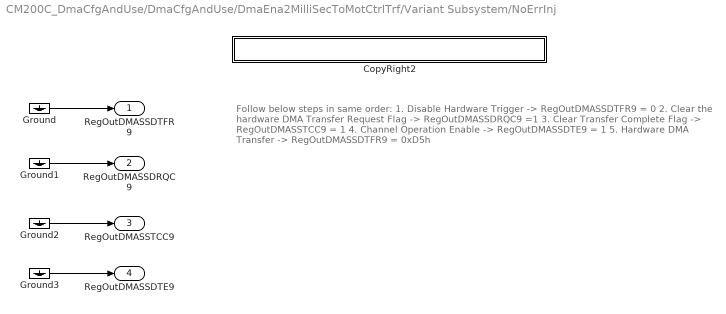
== system CM200C_DmaCfgAndUse/DmaCfgAndUse/DmaEna2MilliSecToMotCtrlTrf/Variant Subsystem/NoErrInj ==
  note: Follow below steps in same order:
      |
      | 1. Disable Hardware Trigger -> RegOutDMASSDTFR9 = 0
      | 2. Clear the hardware DMA Transfer Request Flag -> RegOutDMASSDRQC9 =1
      | 3. Clear Transfer Complete Flag -> RegOutDMASSTCC9 = 1
      | 4. Channel Operation Enable -> RegOutDMASSDTE9 = 1
      | 5. Hardware DMA Transfer -> RegOutDMASSDTFR9 = 0xD5h
  CopyRight2 : Subsystem  Description=|  mask(Copyright Information){none=on}
      | Copyright info block.                                               
      |                                                                     
      | Place copyright information at the top of every subsystem in design.
      mask prompts: none "No parameters"
      mask help: Place copyright information at the top of every subsystem in design.
      mask Display:
      | NxtrConf = 'Nexteer Confidential';
      | 
      | sys = bdroot; %handle for the current model ("system")
      | first = get_param(sys,'Created');
      | first = first(end-3:end);  %year is last four digits
      | 
      | last = get_param(sys,'LastModifiedDate');
      | if isempty(last)
      |     last = datestr(now,'yyyy');
      | else
      |     last = last(end-3:end);
      | end
      | 
      | if strcmp(first,last)
      |     fprintf('%s -- Copyright %s Nexteer',NxtrConf,first)
      | else
      |     fprintf('%s -- %s%s- %s Nexteer',NxtrConf,char(169),first,last)
      | end
  Ground{,1..3} (4 alike) : Ground
  RegOutDMASSDTFR9 : Outport
  RegOutDMASSDRQC9 : Outport  Port=2
  RegOutDMASSTCC9 : Outport  Port=3
  RegOutDMASSDTE9 : Outport  Port=4
  wires:
  Ground3/1 -> RegOutDMASSDTE9/1
  Ground2/1 -> RegOutDMASSTCC9/1
  Ground1/1 -> RegOutDMASSDRQC9/1
  Ground/1 -> RegOutDMASSDTFR9/1

== system CM200C_DmaCfgAndUse/DmaCfgAndUse/DmaWaitForMotCtrlTo2MilliSecTrf/GetTiSpan1MicroSec32bit/CopyRight2 ==

== system CM200C_DmaCfgAndUse/DmaCfgAndUse/DmaWaitForMotCtrlTo2MilliSecTrf/If Action Subsystem/CopyRight2 ==

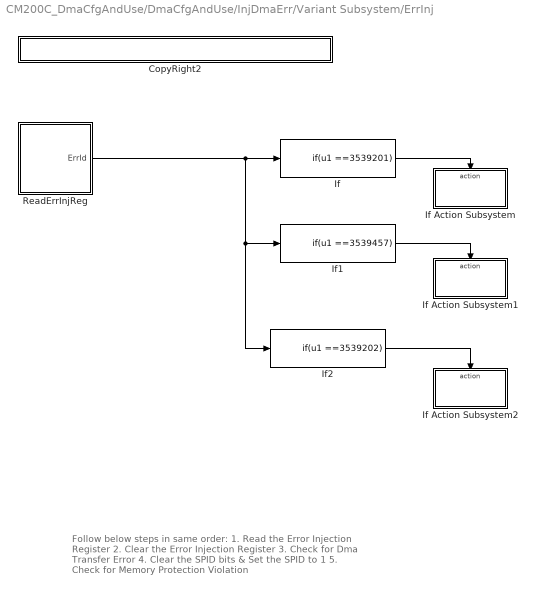
== system CM200C_DmaCfgAndUse/DmaCfgAndUse/InjDmaErr/Variant Subsystem/ErrInj ==
  note: Follow below steps in same order:
      |
      | 1. Read the Error Injection Register
      | 2. Clear the Error Injection Register
      | 3. Check for Dma Transfer Error
      | 4. Clear the SPID bits & Set the SPID to 1
      | 5. Check for Memory Protection Violation
  CopyRight2 : Subsystem  Description=|  mask(Copyright Information){none=on}
      | Copyright info block.                                               
      |                                                                     
      | Place copyright information at the top of every subsystem in design.
      mask prompts: none "No parameters"
      mask help: Place copyright information at the top of every subsystem in design.
      mask Display:
      | NxtrConf = 'Nexteer Confidential';
      | 
      | sys = bdroot; %handle for the current model ("system")
      | first = get_param(sys,'Created');
      | first = first(end-3:end);  %year is last four digits
      | 
      | last = get_param(sys,'LastModifiedDate');
      | if isempty(last)
      |     last = datestr(now,'yyyy');
      | else
      |     last = last(end-3:end);
      | end
      | 
      | if strcmp(first,last)
      |     fprintf('%s -- Copyright %s Nexteer',NxtrConf,first)
      | else
      |     fprintf('%s -- %s%s- %s Nexteer',NxtrConf,char(169),first,last)
      | end
  If : If  Description=ErrId - 0x00360101  IfExpression=u1 ==3539201  ShowElse=off
      settings: AttributesFormatString=|
      | %<IfExpression>
      | %<Description>
  If Action Subsystem : Subsystem  TreatAsAtomicUnit=on
  If Action Subsystem1 : Subsystem  TreatAsAtomicUnit=on
  If Action Subsystem2 : Subsystem  TreatAsAtomicUnit=on
  If1 : If  Description=ErrId - 0x00360201  IfExpression=u1 ==3539457  ShowElse=off
      settings: AttributesFormatString=|
      | %<IfExpression>
      | %<Description>
  If2 : If  Description=ErrId - 0x00360102  IfExpression=u1 ==3539202  ShowElse=off
      settings: AttributesFormatString=|
      | %<IfExpression>
      | %<Description>
  ReadErrInjReg : Subsystem
      settings: AttributesFormatString=Client Call : Read the Fault Injection Register
  wires:
  ReadErrInjReg/1(ErrId) -> If2/1, If1/1, If/1
  If/1 -> If Action Subsystem/Action
  If1/1 -> If Action Subsystem1/Action
  If2/1 -> If Action Subsystem2/Action

== system CM200C_DmaCfgAndUse/DmaCfgAndUse/InjMcuDiagcErr/Variant Subsystem/ErrInj ==
  note: Follow below steps in same order:
      |
      | 1. Read the Error Injection Register
      | 2. Check for Dma Transfer Error
      |    2a. Clear the Error Injection Register
      |    2b. Clear the DMASSDCEN15
  Action : Subsystem  TreatAsAtomicUnit=on
  CopyRight2 : Subsystem  Description=|  mask(Copyright Information){none=on}
      | Copyright info block.                                               
      |                                                                     
      | Place copyright information at the top of every subsystem in design.
      mask prompts: none "No parameters"
      mask help: Place copyright information at the top of every subsystem in design.
      mask Display:
      | NxtrConf = 'Nexteer Confidential';
      | 
      | sys = bdroot; %handle for the current model ("system")
      | first = get_param(sys,'Created');
      | first = first(end-3:end);  %year is last four digits
      | 
      | last = get_param(sys,'LastModifiedDate');
      | if isempty(last)
      |     last = datestr(now,'yyyy');
      | else
      |     last = last(end-3:end);
      | end
      | 
      | if strcmp(first,last)
      |     fprintf('%s -- Copyright %s Nexteer',NxtrConf,first)
      | else
      |     fprintf('%s -- %s%s- %s Nexteer',NxtrConf,char(169),first,last)
      | end
  If : If  Description=ErrId - 0x002B0101  IfExpression=u1 ==2818305  ShowElse=off
      settings: AttributesFormatString=|
      | %<IfExpression>
      | %<Description>
  ReadErrInjReg : Subsystem
      settings: AttributesFormatString=Client Call : Read the Fault Injection Register
  wires:
  ReadErrInjReg/1(ErrId) -> If/1
  If/1 -> Action/Action

== system CM200C_DmaCfgAndUse/DmaCfgAndUse/DmaEna2MilliSecToMotCtrlTrf/Variant Subsystem/ErrInj/CopyRight2 ==

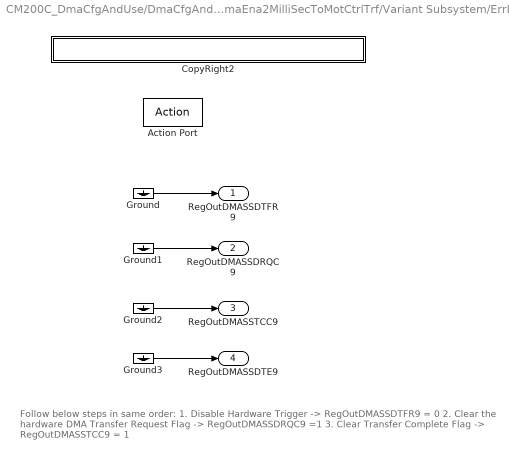
== system CM200C_DmaCfgAndUse/DmaCfgAndUse/DmaEna2MilliSecToMotCtrlTrf/Variant Subsystem/ErrInj/If Action Subsystem ==
  note: Follow below steps in same order:
      |
      | 1. Disable Hardware Trigger -> RegOutDMASSDTFR9 = 0
      | 2. Clear the hardware DMA Transfer Request Flag -> RegOutDMASSDRQC9 =1
      | 3. Clear Transfer Complete Flag -> RegOutDMASSTCC9 = 1
  Action Port : ActionPort
  CopyRight2 : Subsystem  Description=|  mask(Copyright Information){none=on}
      | Copyright info block.                                               
      |                                                                     
      | Place copyright information at the top of every subsystem in design.
      mask prompts: none "No parameters"
      mask help: Place copyright information at the top of every subsystem in design.
      mask Display:
      | NxtrConf = 'Nexteer Confidential';
      | 
      | sys = bdroot; %handle for the current model ("system")
      | first = get_param(sys,'Created');
      | first = first(end-3:end);  %year is last four digits
      | 
      | last = get_param(sys,'LastModifiedDate');
      | if isempty(last)
      |     last = datestr(now,'yyyy');
      | else
      |     last = last(end-3:end);
      | end
      | 
      | if strcmp(first,last)
      |     fprintf('%s -- Copyright %s Nexteer',NxtrConf,first)
      | else
      |     fprintf('%s -- %s%s- %s Nexteer',NxtrConf,char(169),first,last)
      | end
  Ground{,1..3} (4 alike) : Ground
  RegOutDMASSDTFR9 : Outport
  RegOutDMASSDRQC9 : Outport  Port=2
  RegOutDMASSTCC9 : Outport  Port=3
  RegOutDMASSDTE9 : Outport  Port=4
  wires:
  Ground3/1 -> RegOutDMASSDTE9/1
  Ground2/1 -> RegOutDMASSTCC9/1
  Ground1/1 -> RegOutDMASSDRQC9/1
  Ground/1 -> RegOutDMASSDTFR9/1

== system CM200C_DmaCfgAndUse/DmaCfgAndUse/DmaEna2MilliSecToMotCtrlTrf/Variant Subsystem/ErrInj/ReadErrInjReg ==
  CopyRight2 : Subsystem  Description=|  mask(Copyright Information){none=on}
      | Copyright info block.                                               
      |                                                                     
      | Place copyright information at the top of every subsystem in design.
      mask prompts: none "No parameters"
      mask help: Place copyright information at the top of every subsystem in design.
      mask Display:
      | NxtrConf = 'Nexteer Confidential';
      | 
      | sys = bdroot; %handle for the current model ("system")
      | first = get_param(sys,'Created');
      | first = first(end-3:end);  %year is last four digits
      | 
      | last = get_param(sys,'LastModifiedDate');
      | if isempty(last)
      |     last = datestr(now,'yyyy');
      | else
      |     last = last(end-3:end);
      | end
      | 
      | if strcmp(first,last)
      |     fprintf('%s -- Copyright %s Nexteer',NxtrConf,first)
      | else
      |     fprintf('%s -- %s%s- %s Nexteer',NxtrConf,char(169),first,last)
      | end
  Ground : Ground
  ErrId : Outport
  wires:
  Ground/1 -> ErrId/1

== system CM200C_DmaCfgAndUse/DmaCfgAndUse/DmaEna2MilliSecToMotCtrlTrf/Variant Subsystem/NoErrInj/CopyRight2 ==

== system CM200C_DmaCfgAndUse/DmaCfgAndUse/InjDmaErr/Variant Subsystem/ErrInj/CopyRight2 ==
